simulink model "FullOrderObserver"  (R2024b)
settings: Solver=ode45  StartTime=0.0  StopTime=inf  MaxStep=5e-6  RelTol=1e-3  EnableMultiTasking=on
InitFcn:
  | %电机参数
  | Pe=4000; Ve=380; fe=50;
  | Rs=1.087; Rr=0.788;
  | Ls=0.148; Lr=0.148; Lm=0.140;
  | J=0.0131;FF=0.002985; np=2;
  | %其他参数
  | Ts=5e-6;
  | fs=5000;
  | Udc=540;
  | k=1.5;
undefined symbols (not defined in the file): DiscIntNeverNeededParam, spd
libraries: powerlib_extras x3, spsDCVoltageSourceLib x2, spsAsynchronousMachineSIUnitsLib x1, spsGroundLib x1, simulink x1, spsThreePhaseVIMeasurementLib x1, spsUniversalBridgeLib x1, sps_lib x1
settings Model: Creator=Lenovo  LastModifiedBy=SESA504213
settings SolverCC: AlgebraicLoopSolver=TrustRegion
settings DataIOCC: LimitDataPoints=on  SaveFormat=Array  SignalLoggingSaveFormat=ModelDataLogs  ReturnWorkspaceOutputs=off
settings OptimizationCC: ExpressionDepthLimit=2147483647  LifeSpan=inf
settings DebuggingCC: UnderspecifiedInitializationDetection=Classic  MergeDetectMultiDrivingBlocksExec=none  SolverPrmCheckMsg=warning  FcnCallInpInsideContextMsg=warning  UnconnectedInputMsg=warning  UnconnectedOutputMsg=warning  UnconnectedLineMsg=warning  StateNameClashWarn=warning  SFUnexpectedBacktrackingDiag=warning  SFNoUnconditionalDefaultTransitionDiag=warning  SFExecutionAtInitializationDiag=none  ArithmeticOperatorsInVariantConditions=warning
settings HardwareCC: ProdBitPerPointer=32  ProdBitPerSizeT=32  ProdBitPerPtrDiffT=32  ProdLargestAtomicFloat=None  ProdIntDivRoundTo=Undefined  ProdEndianess=Unspecified  ProdWordSize=32  ProdHWDeviceType=32-bit Generic
settings ModelReferenceCC: EnableRefExpFcnMdlSchedulingChecks=on  PropagateSignalLabelsOutOfModel=off
settings SFSimCC: SimUseLocalCustomCode=off  CustomCodeUndefinedFunction=UseInterfaceOnly
settings RTWCC: RTWUseLocalCustomCode=off  GPUComputeCapability=3.5
settings CodeAppCC: StateflowObjectComments=on
settings GRTTargetCC: TargetLangStandard=C89/C90 (ANSI)  CombineOutputUpdateFcns=off  GRTInterface=on
settings ConfigComp: CovMetricSettings=dw  CovSaveCumulativeToWorkspaceVar=on  CovSaveSingleToWorkspaceVar=on  CovExternalEMLEnable=off

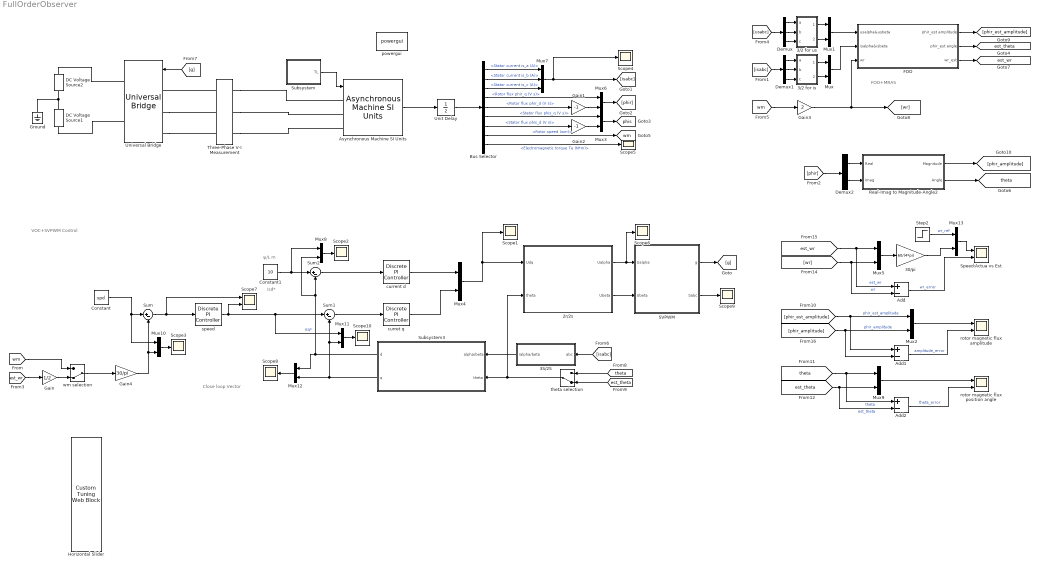
== system FullOrderObserver ==
  note: FOO+MRAS
  note: VOC+SVPWM Control
  note: Close loop Vector
  note: ψ/L m
  note: isd*
  " rotor magnetic flux amplitude" : Scope  NumInputPorts=2
  2r/2s : Subsystem
  3/2 for is : Subsystem
  3/2 for us : Subsystem
  30/pi : Gain  Gain=60/(4*pi)
  3S/2S : Subsystem
  Add : Sum  Inputs=+-
  Add1 : Sum  Inputs=+-
  Add2 : Sum  Inputs=+-
  Asynchronous Machine SI Units : spsAsynchronousMachineSIUnitsLib/Asynchronous Machine SI Units  RotorType=Squirrel-cage  PresetModel=No  MechanicalLoad=Torque Tm  ShowDetailedParameters=on  ReferenceFrame=Stationary  Units=SI  MeasurementBus=off  NominalParameters=[Pe Ve fe]  VoltageRatio=1  Stator=[Rs Ls-Lm]  Rotor=[Rr Lr-Lm]  Cage1=[ 0.022 0.226/377]  Cage2=[ 0.022 0.226/377]  Lm=Lm  Mechanical=[J FF np]  PolePairs=2  InitialConditions=[1 0 0 0 0 0 0 0]  SimulateSaturation=off  Saturation=[14.03593122, 27.81365428, 53.79336849, 72.68890987, 97.98006896, 148.6815601, 215.7428561, 302.9841135, 420.4778367 ; 230, 322, 414, 460, 506, 552, 598, 644, 690]  LoadFlowParameters=1492000  TsPowergui=0  TsBlock=-1  IterativeModel=Forward Euler  IterativeDiscreteModel=Trapezoidal non iterative  Pmec=1.492e+006
      settings: AttributesFormatString=\n
  Bus Selector : BusSelector  OutputSignals=Stator measurements.Stator current is_a (A),Stator measurements.Stator current is_b (A),Stator measurements.Stator current is_c (A),Rotor measurements.Rotor flux phir_q (V s),Rotor measurements.Rotor flux phir_d (V s),Stator measurements.Stator flux phis_q (V s),Stator measurements.Stator flux phis_d (V s),Mechanical.Rotor speed (wm),Mechanical.Electromagnetic torque Te (N*m)
  Constant : Constant  Value=spd
  Constant1 : Constant  Value=10  SampleTime=0
  DC Voltage Source1 : spsDCVoltageSourceLib/DC Voltage Source  Amplitude=Udc/2  Measurements=None
  DC Voltage Source2 : spsDCVoltageSourceLib/DC Voltage Source  Amplitude=Udc/2  Measurements=None
  Demux : Demux  Outputs=3
  Demux1 : Demux  Outputs=3
  Demux2 : Demux  Outputs=2
  FOO : Subsystem
  Gain : Gain  Gain=1/2
  Gain1 : Gain  Gain=-1
  Gain2 : Gain  Gain=-1
  Gain3 : Gain  Gain=2
  Gain4 : Gain  Gain=30/pi
  Ground : spsGroundLib/Ground  LConnTagsString=a
  Horizontal Slider : CustomTuningWebBlock  LabelPosition=Hide  ShowInitialText=on  Configuration="{\"components\":[{\"name\":\"LinearScaleComponent\",\"settings\":{\"bounds\":{\"max\":3000,\"min\":0,\"tickInterval\":\"auto\"},\"internalTickHeightScaleFactor\":0.5,\"labelColor\":[255,255,200],\"labelFont\":{\"font\":\"Arial\",\"fontSize\":12},\"labelOffset\":0.05,\"labelTransparency\":1,\"needleImage\":{\"size\":[596,842],\"src\":\"data:image\\/svg+xml;base64,PD94bWwgdmVyc2lvbj0iMS4wIiBlbmNvZGluZz0idXRmLTgiPz4NCjwhLS0gR2VuZXJhdG9yOiBBZG9iZSBJbGx1c3RyYXRvciAyNS4wLjAsIFNWRyBFeHBvcnQgUGx1Zy1JbiAuIFNWRyBWZXJzaW9uOiA2LjAwIEJ1aWxkIDApICAtLT4NCjxzdmcgdmVyc2lvbj0iMS4xIg0KCSBpZD0ic3ZnOCIgeG1sbnM6Y2M9Imh0dHA6Ly9jcmVhdGl2ZWNvbW1vbnMub3JnL25zIyIgeG1sbnM6ZGM9Imh0dHA6Ly9wdXJsLm9yZy9kYy9lbGVtZW50cy8xLjEvIiB4bWxuczppbmtzY2FwZT0iaHR0cDovL3d3dy5pbmtzY2FwZS5vcmcvbmFtZXNw ...(+2420 chars)\",\"srcOrientation\":\"Right\"},\"needleOffset\":[0.0642123287671233,-0.8044596912521441],\"needleSize\":{\"height\":0.07668067226890757,\"width\":0.4337797619047619},\"position\":[0.03637079831932777,0.2829861111111111,0.6088789682539683,0.9196428571428571],\"referencePoint\":\"auto\",\"scaleColors\":[],\"scaleColorsSize\":0.2,\"scaleDirection\":\"BT\",\"showLabels\":1,\"showMinorTicks\":0,\"showSpanLine\":1,\"showTicks\":1,\"tickColor\":[252,252,197],\"tickTransparency\":1,\"valueBarColor\":[0,114,189],\"valueBarOffset\":-0.27,\"valueBarSize\":0.1,\"valueBarTransparency\":1}},{\"name\":\"BackgroundImageComponent\",\"settings\":{\"image\":{\"size\":[380,101],\"src\":\"data:image\\/svg+xml;base64,PHN2ZyB4bWxucz0iaHR0cDovL3d3dy53My5vcmcvMjAwMC9zdmciIHhtbG5zOnhsaW5rPSJodHRwOi8vd3d3LnczLm9yZy8xOTk5L3hsaW5rIiB2aWV3Qm94PSIwIDAgMzgwIDEwMSI+PGRlZnM+PHN0eWxlPi5jbHMtMXtmaWxsOiMwMDJiNDI7fS5jbHMtMntmaWxsOiM0MjcwODI7fS5jbHMtM3tmaWxsOnVybCgjcmFkaWFsLWdyYWRpZW50KTt9LmNscy00e2ZpbGw6I2M4YzhjODtzdHJva2U6IzAwMDt9PC9zdHlsZT48cmFkaWFsR3JhZGllbnQgaWQ9InJhZGlhbC1ncmFkaWVudCIgY3g9IjE5MCIgY3k9IjUwLjUiIHI9IjI2OS4yMSIgZ3JhZGllbnRVbml0cz0idXNlclNwYWNlT25Vc2UiPjxzdG9wIG9mZnNldD0iMC4wMSIgc3RvcC1jb2xvcj0iIzNlNGY1OCIvPjxzdG9wIG9mZnNldD0iMC4wNiIgc3RvcC1jb2xvcj0iIzQ0NTc2MSIvPjxzdG9wIG9mZnNldD0iMC4xNSIgc3RvcC1jb2xvcj0iIzU1NmE3NiIvPjxzdG9wIG9mZnNldD0iMC4yNSIgc3RvcC1jb2xvcj0iIzZkODg5NSIvPjxzdG9wIG9mZnNldD0iMC4zOCIgc3RvcC1jb2xvcj0iIzhmYjJjMyIvPjxzdG9wIG9mZnNldD0iMC41MiIgc3RvcC1jb2xvcj0iI2I2ZTRmYSIvPjxzdG9wIG9mZnNldD0iMSIgc3RvcC1jb2xvcj0iIzE1NDY1NyIvPjwvcmFkaWFsR3JhZGllbnQ+PC9kZWZzPjxnIGlkPSJmcmFtZSI+PGcgaWQ9IkxheWVyXzIiIGRhdGEtbmFtZT0iTGF5ZXIgMiI+PGcgaWQ9IkxheWVyXzEtMiIgZGF0YS1uYW1lPSJMYXllciAxLTIiPjxyZWN0IGlkPSJyZWN0MTAzNiIgY2xhc3M9ImNscy0xIiB4PSIxMSIgeT0iMTEiIHdpZHRoPSIzNTgiIGhlaWdodD0iNzkiLz48cGF0aCBpZD0icGF0aDEwMzgiIGNsYXNzPSJjbHMtMiIgZD0iTTgsOFY5M0gzNzJWOFpNMzY5LDkwSDExVjExSDM2OVoiLz48cGF0aCBpZD0icGF0aDEwNDAiIGNsYXNzPSJjbHMtMyIgZD0iTTAsMFYxMDFIMzgwVjBaTTM3Miw5M0g4VjhIMzcyWiIvPjwvZz48L2c+PC9nPjxnIGlkPSJ0cmFjayI+PHBhdGggaWQ9InJlY3QxNjExIiBjbGFzcz0iY2xzLTQiIGQ9Ik0zMy4zNywyNi41OUgzNDYuNjNjNCwwLDcuMjUsMi42LDcuMjUsNS44MWgwYzAsMy4yMS0zLjI1LDUuODItNy4yNSw1LjgySDMzLjM3Yy00LDAtNy4yNS0yLjYxLTcuMjUtNS44MmgwQzI2LjEyLDI5LjE5LDI5LjM3LDI2LjU5LDMzLjM3LDI2LjU5WiIvPjwvZz48L3N2Zz4=\",\"srcOrientation\":\"horizontal\"},\"position\":[0,0,1,1],\"scaleMode\":\"0\"}},{\"name\":\"ForegroundImageComponent\",\"settings\":{\"image\":{\"size\":[0,0],\"src\":\"default\",\"srcOrientation\":[]},\"isForeground\":1,\"position\":[0,0,1,1],\"scaleMode\":\"0\"}}],\"settings\":{\"BindingType\":\"param\",\"aspectRatio\":3.7777777777777777,\"backgroundColor\":[0,0,0,\"1\"],\"backgroundOffset\":0,\"backgroundOpacity\":1,\"fixedAspectRatio\":\"on\",\"foregroundColor\":[252,252,196],\"orientation\":\"vertical\",\"showBackgroundColor\":false,\"value\":0,\"version\":\"R2023a\"},\"type\":\"LinearGauge\"}"
  Mux{,1..6,8..13} (13 alike) : Mux  Inputs=2
  Mux7 : Mux  Inputs=3
  Real-Imag to Magnitude-Angle2 : Subsystem
  SVPWM : Subsystem
  Scope{1..6,8..10} (9 alike) : Scope
  Scope7 : Scope  NumInputPorts=2
  Speed:Actua vs Est : Scope  NumInputPorts=2
  Step2 : Step  Before=500  After=1000  SampleTime=0
  Subsystem : Subsystem
  Subsystem3 : Subsystem
  Sum : Sum  Inputs=|+-
  Sum1 : Sum  Inputs=|+-
  Sum2 : Sum  Inputs=|+-
  Three-Phase V-I Measurement : spsThreePhaseVIMeasurementLib/Three-Phase V-I Measurement  VoltageMeasurement=phase-to-ground  SetLabelV=on  LabelV=usabc  Vpu=off  VpuLL=off  CurrentMeasurement=no  SetLabelI=off  LabelI=Iabc  Ipu=off  Pbase=100e6  Vbase=500e3  OutputType=Complex  PhasorSimulation=off  PSBequivalent=0
  Unit Delay : UnitDelay  SampleTime=-1
  Universal Bridge : spsUniversalBridgeLib/Universal Bridge  Arms=3  SnubberResistance=1e5  SnubberCapacitance=inf  Device=IGBT / Diodes  Ron=1e-3  Lon=0  ForwardVoltages="[  0  0  ]"  ForwardVoltage=0  GTOparameters=[ 10e-6 , 20e-6 ]  IGBTparameters=[ 1e-6 , 2e-6]  Measurements=Device voltages  Measurements_2=None  converterType=Rectifier
  current d : powerlib_extras/Discrete  Control Blocks/Discrete PI Controller  Kp=15*15  Ki=600*2  Par_Limits=[310*1.5 -310*1.5]  Init=0  Ts=-1
  curret q : powerlib_extras/Discrete  Control Blocks/Discrete PI Controller  Kp=15*15  Ki=600*2  Par_Limits=[310*1.5 -310*1.5]  Init=0  Ts=-1
  powergui : sps_lib/powergui  Priority=1  SimulationMode=Discrete  SampleTime=5e-6  frequency=60  Iterations=50  frequencyindice=50  Pbase=100e6  ErrMax=1e-4  UnitsV=kV  UnitsW=MW  buscounter=0  FunctionMessages=off  echomessages=off  EnableUseOfTLC=off  CurrentSourceSwitches=off  DisableSnubberDevices=off  DisableRonSwitches=off  DisableVfSwitches=off  DisplayEquations=off  AutomaticDiscreteSolvers=off  SolverType=Tustin/Backward Euler (TBE)  Interpol=off  ExternalGateDelay=off  methode=off  Ts=0  x0status=blocks  SPID=off  SwTol=0  HookPort=off  NonlinearTolerance=1e-4  nMaxIteration=100  ContinueOnMaxIteration=off  RestoreLinks=warning  ResistiveCurrentMeasurement=off  Frange=[0:2:500]  Ylog=off  Xlog=on  ShowGrid=off  save=off  variable=ZData  structure=0  ZoomFFT=off  StartTime=0.0  cycles=1  DisplayStyle=1  fundamental=60  FreqAxis=off  MaxFrequency=1000  frequencyindicesteady=1  RmsSteady=1  display=off
  "rotor magnetic flux position angle " : Scope  NumInputPorts=2
  speed : powerlib_extras/Discrete  Control Blocks/Discrete PI Controller  Kp=0.4  Ki=15  Par_Limits=[30 -30]  Init=0  Ts=-1
  theta selection : ManualSwitch  CurrentSetting=0
  wm selection : ManualSwitch  CurrentSetting=0
  tag scope: est_theta=global, est_wr=global, phis=global, theta=global, wm=global
  wires:
  Bus Selector/1 -> Mux7/1  "<Stator current is_a (A)>"
  Bus Selector/2 -> Mux7/2  "<Stator current is_b (A)>"
  Bus Selector/3 -> Mux7/3  "<Stator current is_c (A)>"
  Gain2/1 -> Mux3/2
  Mux2/1 -> " rotor magnetic flux amplitude"/1
  Mux5/1 -> 30/pi/1
  Demux2/1 -> Real-Imag to Magnitude-Angle2/1(Real)
  Demux2/2 -> Real-Imag to Magnitude-Angle2/2(Imag)
  Bus Selector/7 -> Gain2/1  "<Stator flux phis_d (V s)>"
  Bus Selector/6 -> Mux3/1  "<Stator flux phis_q (V s)>"
  [isabc] -> Demux1/1
  Demux1/1 -> 3/2 for is/1(a)
  Demux1/2 -> 3/2 for is/2(b)
  Demux1/3 -> 3/2 for is/3(c)
  3/2 for is/1(alpha) -> Mux/1
  3/2 for is/2(beta) -> Mux/2
  Gain1/1 -> Mux6/2
  Bus Selector/5 -> Gain1/1  "<Rotor flux phir_d (V s)>"
  Bus Selector/4 -> Mux6/1  "<Rotor flux phir_q (V s)>"
  Mux6/1 -> [phir]
  Mux3/1 -> [phis]
  [usabc] -> Demux/1
  Demux/1 -> 3/2 for us/1(a)
  Demux/2 -> 3/2 for us/2(b)
  Demux/3 -> 3/2 for us/3(c)
  3/2 for us/1(alpha) -> Mux1/1
  3/2 for us/2(beta) -> Mux1/2
  Mux1/1 -> FOO/1(usalpha&usbeta)
  Mux/1 -> FOO/2(isalpha&isbeta)
  Bus Selector/8 -> [wm]  "<Rotor speed (wm)>"
  [wm] -> Gain3/1
  Mux9/1 -> "rotor magnetic flux position angle "/1
  [phir] -> Demux2/1
  FOO/2(phir_est angle) -> [est_theta]
  Gain3/1 -> [wr], FOO/3("wr ")
  Bus Selector/9 -> Scope5/1  "<Electromagnetic torque Te (N*m)>"
  FOO/3(wr_est) -> [est_wr]
  30/pi/1 -> Mux13/2
  Real-Imag to Magnitude-Angle2/2(Angle) -> [theta]
  Mux7/1 -> [isabc], Scope4/1
  SVPWM/1(g) -> [g]
  [g] -> Universal Bridge/1
  [wm] -> wm selection/1
  [theta] -> theta selection/1
  [est_theta] -> theta selection/2
  Asynchronous Machine SI Units/1 -> Unit Delay/1
  Unit Delay/1 -> Bus Selector/1
  Gain/1 -> wm selection/2
  [est_wr] -> Gain/1
  wm selection/1 -> Gain4/1
  theta selection/1 -> Subsystem3/2(theta), 2r/2s/2(theta)
  SVPWM/2(Sabc) -> Scope9/1
  speed/1 -> Sum1/1, Mux11/1, Scope7/2  "isq*"
  Constant/1 -> Mux10/1, Sum/1
  Sum/1 -> Scope7/1, speed/1
  Sum2/1 -> current d/1
  curret q/1 -> Mux4/2
  current d/1 -> Mux4/1
  Mux11/1 -> Scope10/1
  Mux10/1 -> Scope3/1
  Mux12/1 -> Scope8/1
  Mux8/1 -> Scope2/1
  Gain4/1 -> Mux10/2, Sum/2
  Sum1/1 -> curret q/1
  Mux4/1 -> Scope1/1, 2r/2s/1(Udq)
  2r/2s/2(Ubeta) -> SVPWM/2(Ubeta)
  2r/2s/1(Ualpha) -> Scope6/1, SVPWM/1(Ualpha)
  Subsystem3/2(q) -> Sum1/2, Mux11/2, Mux12/2
  Subsystem3/1(d) -> Mux12/1, Sum2/2, Mux8/2
  3S/2S/1(ialpha/beta) -> Subsystem3/1(alpha/beta)
  [isabc] -> 3S/2S/1(abc)
  Constant1/1 -> Mux8/1, Sum2/1
  Add/1 -> Speed:Actua vs Est/2  "wr_error"
  [est_wr] -> Mux5/1, Add/1  "est_wr"
  [theta] -> Mux9/1, Add2/1  "theta"
  [est_theta] -> Mux9/2, Add2/2  "est_theta"
  [wr] -> Mux5/2, Add/2  "wr"
  FOO/1(phir_est amplitude) -> [phir_est_amplitude]
  Real-Imag to Magnitude-Angle2/1(Magnitude) -> [phir_amplitude]
  [phir_amplitude] -> Mux2/2, Add1/2  "phir_amplitude"
  Add1/1 -> " rotor magnetic flux amplitude"/2  "amplitude_error"
  Add2/1 -> "rotor magnetic flux position angle "/2  "theta_error"
  Step2/1 -> Mux13/1  "wr_ref"
  Mux13/1 -> Speed:Actua vs Est/1
  [phir_est_amplitude] -> Add1/1, Mux2/1  "phir_est_amplitude"
  Subsystem/1(TL) -> Asynchronous Machine SI Units/1
  connections:
  DC Voltage Source1/RConn1 -- Ground/LConn1 -- DC Voltage Source2/LConn1
  DC Voltage Source1/LConn1 -- Universal Bridge/RConn2
  Three-Phase V-I Measurement/RConn2 -- Asynchronous Machine SI Units/LConn2
  Three-Phase V-I Measurement/RConn1 -- Asynchronous Machine SI Units/LConn1
  Three-Phase V-I Measurement/LConn1 -- Universal Bridge/LConn1
  Universal Bridge/LConn2 -- Three-Phase V-I Measurement/LConn2
  Universal Bridge/LConn3 -- Three-Phase V-I Measurement/LConn3
  Three-Phase V-I Measurement/RConn3 -- Asynchronous Machine SI Units/LConn3
  DC Voltage Source2/RConn1 -- Universal Bridge/RConn1

== system FullOrderObserver/2r//2s ==
  Udq : Inport
  theta : Inport  Port=2
  Demux : Demux  Outputs=2
  Mux1 : Mux  Inputs=2
  Product{,1..3} (4 alike) : Product  RndMeth=Zero
  Scope1 : Scope
  Sum : Sum  Inputs=|+-
  Sum1 : Sum  Inputs=|++
  Trigonometric Function : Trigonometry
  Trigonometric Function1 : Trigonometry  Operator=cos
  Ualpha : Outport
  Ubeta : Outport  Port=2
  wires:
  Udq/1 -> Demux/1
  Product/1 -> Sum/1
  Product1/1 -> Sum/2
  Product2/1 -> Sum1/1
  Product3/1 -> Sum1/2
  Sum/1 -> Ualpha/1, Mux1/1
  Sum1/1 -> Ubeta/1, Mux1/2
  Demux/1 -> Product/1, Product2/1
  Trigonometric Function1/1 -> Product/2, Product3/2
  Demux/2 -> Product1/1, Product3/1
  Trigonometric Function/1 -> Product1/2, Product2/2
  theta/1 -> Trigonometric Function/1, Trigonometric Function1/1
  Mux1/1 -> Scope1/1

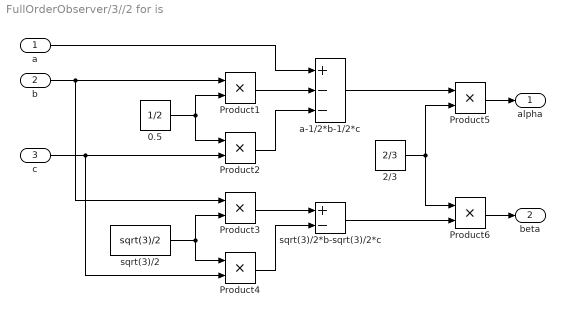
== system FullOrderObserver/3//2 for is ==
  a : Inport
  b : Inport  Port=2
  c : Inport  Port=3
  0.5 : Constant  Value=1/2
  2/3 : Constant  Value=2/3
  Product{1..6} (6 alike) : Product  RndMeth=Zero
  a-1/2*b-1/2*c : Sum  Inputs=+--
  sqrt(3)/2 : Constant  Value=sqrt(3)/2
  sqrt(3)/2*b-sqrt(3)/2*c : Sum  Inputs=+-
  alpha : Outport
  beta : Outport  Port=2
  wires:
  0.5/1 -> Product1/2, Product2/1
  sqrt(3)/2/1 -> Product3/2, Product4/1
  b/1 -> Product1/1, Product3/1
  c/1 -> Product2/2, Product4/2
  Product1/1 -> a-1/2*b-1/2*c/2
  Product2/1 -> a-1/2*b-1/2*c/3
  a/1 -> a-1/2*b-1/2*c/1
  Product3/1 -> sqrt(3)/2*b-sqrt(3)/2*c/1
  Product4/1 -> sqrt(3)/2*b-sqrt(3)/2*c/2
  a-1/2*b-1/2*c/1 -> Product5/1
  2/3/1 -> Product5/2, Product6/1
  sqrt(3)/2*b-sqrt(3)/2*c/1 -> Product6/2
  Product5/1 -> alpha/1
  Product6/1 -> beta/1

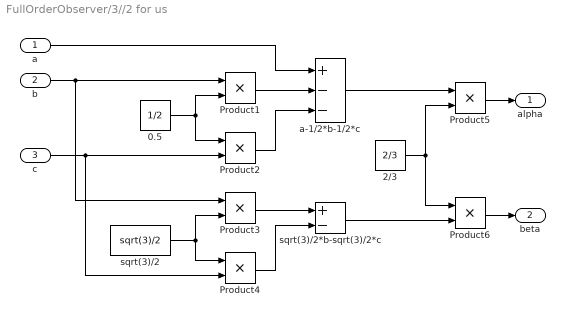
== system FullOrderObserver/3//2 for us ==
  a : Inport
  b : Inport  Port=2
  c : Inport  Port=3
  0.5 : Constant  Value=1/2
  2/3 : Constant  Value=2/3
  Product{1..6} (6 alike) : Product  RndMeth=Zero
  a-1/2*b-1/2*c : Sum  Inputs=+--
  sqrt(3)/2 : Constant  Value=sqrt(3)/2
  sqrt(3)/2*b-sqrt(3)/2*c : Sum  Inputs=+-
  alpha : Outport
  beta : Outport  Port=2
  wires:
  Product6/1 -> beta/1
  Product5/1 -> alpha/1
  sqrt(3)/2*b-sqrt(3)/2*c/1 -> Product6/2
  2/3/1 -> Product6/1, Product5/2
  a-1/2*b-1/2*c/1 -> Product5/1
  Product4/1 -> sqrt(3)/2*b-sqrt(3)/2*c/2
  Product3/1 -> sqrt(3)/2*b-sqrt(3)/2*c/1
  a/1 -> a-1/2*b-1/2*c/1
  Product2/1 -> a-1/2*b-1/2*c/3
  Product1/1 -> a-1/2*b-1/2*c/2
  c/1 -> Product4/2, Product2/2
  b/1 -> Product3/1, Product1/1
  sqrt(3)/2/1 -> Product4/1, Product3/2
  0.5/1 -> Product2/1, Product1/2

== system FullOrderObserver/3S//2S ==
  abc : Inport
  Demux : Demux  Outputs=3
  Gai2 : Gain  Gain=-1/2
  Gain1 : Gain  Gain=-1/2
  Gain3 : Gain  Gain=(sqrt(3))/2
  Gain4 : Gain  Gain=(sqrt(3))/2
  Gain5 : Gain  Gain=2/3
  Gain6 : Gain  Gain=2/3
  Mux3 : Mux  Inputs=2
  Sum : Sum  Inputs=|++
  Sum1 : Sum  Inputs=|++
  Sum2 : Sum  Inputs=|-+
  ialpha/beta : Outport
  wires:
  Mux3/1 -> ialpha/beta/1
  Gain5/1 -> Mux3/1
  Gain6/1 -> Mux3/2
  Demux/3 -> Gain4/1, Gai2/1
  Demux/2 -> Gain3/1, Gain1/1
  Demux/1 -> Sum/1
  Sum2/1 -> Gain6/1
  Sum1/1 -> Gain5/1
  Gain3/1 -> Sum2/2
  Gain4/1 -> Sum2/1
  Sum/1 -> Sum1/1
  Gai2/1 -> Sum1/2
  Gain1/1 -> Sum/2
  abc/1 -> Demux/1

== system FullOrderObserver/FOO ==
  usalpha&usbeta : Inport
  isalpha&isbeta : Inport  Port=2
  "wr " : Inport  Port=3
  " Speed-Adaptation" : Subsystem  mask{Kp=15, Ki=5000}
      mask prompts: Kp "Kp="; Ki "Ki="
  Demux : Demux  Outputs=2
  Demux1 : Demux  Outputs=2
  Real-Imag to Magnitude-Angle : Subsystem
  full order flux observer : Subsystem
  wr selection : ManualSwitch  CurrentSetting=0
  phir_est amplitude : Outport
  phir_est angle : Outport  Port=2
  wr_est : Outport  Port=3
  wires:
  " Speed-Adaptation"/1(wr_est) -> wr_est/1, wr selection/2
  full order flux observer/3(phiralpha_est2) -> " Speed-Adaptation"/5(phiralpha_est), full order flux observer/3(phiralpha_est), Real-Imag to Magnitude-Angle/1(Real)
  wr selection/1 -> full order flux observer/9(wr)
  full order flux observer/2(phisbeta_est2) -> full order flux observer/2(phisbeta_est)
  full order flux observer/6(isbeta_est) -> " Speed-Adaptation"/4(isbeta_est)
  full order flux observer/1(phisalpha_est2) -> full order flux observer/1(phisalpha_est)
  full order flux observer/4(phirbeta_est2) -> " Speed-Adaptation"/6(phirbeta_est), full order flux observer/4(phirbeta_est), Real-Imag to Magnitude-Angle/2(Imag)
  full order flux observer/5(isalpha_est) -> " Speed-Adaptation"/3(isalpha_est)
  "wr "/1 -> wr selection/1
  Demux1/2 -> " Speed-Adaptation"/2(isbeta), full order flux observer/8(isbeta)
  Demux/2 -> full order flux observer/6(usbeta)
  Real-Imag to Magnitude-Angle/2(Angle) -> phir_est angle/1
  Real-Imag to Magnitude-Angle/1(Magnitude) -> phir_est amplitude/1
  Demux/1 -> full order flux observer/5(usalpha)
  usalpha&usbeta/1 -> Demux/1
  Demux1/1 -> " Speed-Adaptation"/1(isalpha), full order flux observer/7(isalpha)
  isalpha&isbeta/1 -> Demux1/1

== system FullOrderObserver/Real-Imag to Magnitude-Angle2 ==
  Real : Inport
  Imag : Inport  Port=2
  2*pi : Constant  Value=2*pi  VectorParams1D=off
  Add : Sum
  Complex to Magnitude-Angle : ComplexToMagnitudeAngle
  Real-Imag to Complex : RealImagToComplex
  Switch : Switch  Criteria=u2 > Threshold  SaturateOnIntegerOverflow=off  InputSameDT=off
  Magnitude : Outport
  Angle : Outport  Port=2
  wires:
  Complex to Magnitude-Angle/2 -> Switch/1, Add/1, Switch/2
  Real-Imag to Complex/1 -> Complex to Magnitude-Angle/1
  Imag/1 -> Real-Imag to Complex/2
  2*pi/1 -> Add/2
  Add/1 -> Switch/3
  Real/1 -> Real-Imag to Complex/1
  Switch/1 -> Angle/1
  Complex to Magnitude-Angle/1 -> Magnitude/1

== system FullOrderObserver/SVPWM ==
  Ualpha : Inport
  Ubeta : Inport  Port=2
  Gain1 : Gain  Gain=2500
  Pulse : Subsystem
  SVPWM : Subsystem
  Scope4 : Scope
  Ts : Constant  Value=1/fs
  Udc : Constant  Value=Udc
  g : Outport
  Sabc : Outport  Port=2
  tag scope: N=global
  wires:
  SVPWM/4(N4) -> [N]
  Pulse/2(Sabc) -> Sabc/1
  Udc/1 -> SVPWM/3(Udc)
  Pulse/1(Pulses) -> g/1
  Ubeta/1 -> SVPWM/2(Ubeta)
  Ualpha/1 -> SVPWM/1(Ualfa)
  Ts/1 -> SVPWM/4(Ts)
  Gain1/1 -> Scope4/1
  SVPWM/1(Tcm1) -> Pulse/1(tcm1), Gain1/1
  SVPWM/2(Tcm2) -> Pulse/2(tcm2)
  SVPWM/3(Tcm3) -> Pulse/3(tcm3)

== system FullOrderObserver/Subsystem ==
  Constant : Constant  Value=0
  Manual Switch : ManualSwitch
  Step : Step  Time=0.5  After=2  SampleTime=0
  TL : Outport  VectorParamsAs1DForOutWhenUnconnected=off
  wires:
  Step/1 -> Manual Switch/2
  Constant/1 -> Manual Switch/1
  Manual Switch/1 -> TL/1

== system FullOrderObserver/Subsystem3 ==
  alpha/beta : Inport
  theta : Inport  Port=2
  Demux1 : Demux  Outputs=2
  Product{,1..3} (4 alike) : Product  RndMeth=Zero
  Sum : Sum  Inputs=|++
  Sum1 : Sum  Inputs=|-+
  Trigonometric Function : Trigonometry
  Trigonometric Function1 : Trigonometry  Operator=cos
  d : Outport
  q : Outport  Port=2
  wires:
  alpha/beta/1 -> Demux1/1
  Demux1/1 -> Product2/1, Product/1
  Demux1/2 -> Product3/1, Product1/1
  Sum1/1 -> q/1
  Sum/1 -> d/1
  Product3/1 -> Sum1/2
  Product2/1 -> Sum1/1
  Product1/1 -> Sum/2
  Product/1 -> Sum/1
  Trigonometric Function/1 -> Product2/2, Product1/2
  Trigonometric Function1/1 -> Product3/2, Product/2
  theta/1 -> Trigonometric Function1/1, Trigonometric Function/1

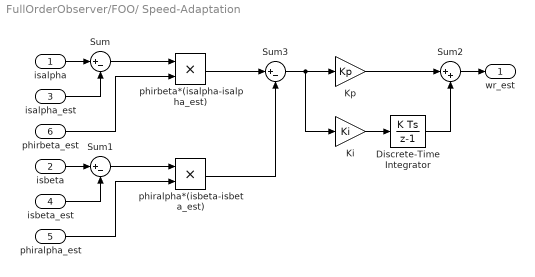
== system FullOrderObserver/FOO/ Speed-Adaptation ==
  isalpha : Inport
  isbeta : Inport  Port=2
  isalpha_est : Inport  Port=3
  isbeta_est : Inport  Port=4
  phiralpha_est : Inport  Port=5
  phirbeta_est : Inport  Port=6
  Discrete-Time Integrator : DiscreteIntegrator  SampleTime=Ts  ICPrevOutput=DiscIntNeverNeededParam  ICPrevScaledInput=DiscIntNeverNeededParam
  Ki : Gain  Gain=Ki
  Kp : Gain  Gain=Kp
  Sum : Sum  Inputs=|+-
  Sum1 : Sum  Inputs=|+-
  Sum2 : Sum  Inputs=|++
  Sum3 : Sum  Inputs=|+-
  phiralpha*(isbeta-isbeta_est) : Product
  phirbeta*(isalpha-isalpha_est) : Product
  wr_est : Outport
  wires:
  Discrete-Time Integrator/1 -> Sum2/2
  Sum/1 -> phirbeta*(isalpha-isalpha_est)/1
  Sum3/1 -> Ki/1, Kp/1
  phiralpha_est/1 -> phiralpha*(isbeta-isbeta_est)/2
  isalpha/1 -> Sum/1
  Sum2/1 -> wr_est/1
  isbeta/1 -> Sum1/1
  phirbeta_est/1 -> phirbeta*(isalpha-isalpha_est)/2
  Sum1/1 -> phiralpha*(isbeta-isbeta_est)/1
  Kp/1 -> Sum2/1
  isalpha_est/1 -> Sum/2
  isbeta_est/1 -> Sum1/2
  phirbeta*(isalpha-isalpha_est)/1 -> Sum3/1
  phiralpha*(isbeta-isbeta_est)/1 -> Sum3/2
  Ki/1 -> Discrete-Time Integrator/1

== system FullOrderObserver/FOO/Real-Imag to Magnitude-Angle ==
  Real : Inport
  Imag : Inport  Port=2
  2*pi : Constant  Value=2*pi  VectorParams1D=off
  Add : Sum
  Complex to Magnitude-Angle : ComplexToMagnitudeAngle
  Real-Imag to Complex : RealImagToComplex
  Switch : Switch  Criteria=u2 > Threshold  SaturateOnIntegerOverflow=off  InputSameDT=off
  Magnitude : Outport
  Angle : Outport  Port=2
  wires:
  Complex to Magnitude-Angle/2 -> Switch/1, Add/1, Switch/2
  Real-Imag to Complex/1 -> Complex to Magnitude-Angle/1
  Imag/1 -> Real-Imag to Complex/2
  2*pi/1 -> Add/2
  Add/1 -> Switch/3
  Real/1 -> Real-Imag to Complex/1
  Switch/1 -> Angle/1
  Complex to Magnitude-Angle/1 -> Magnitude/1

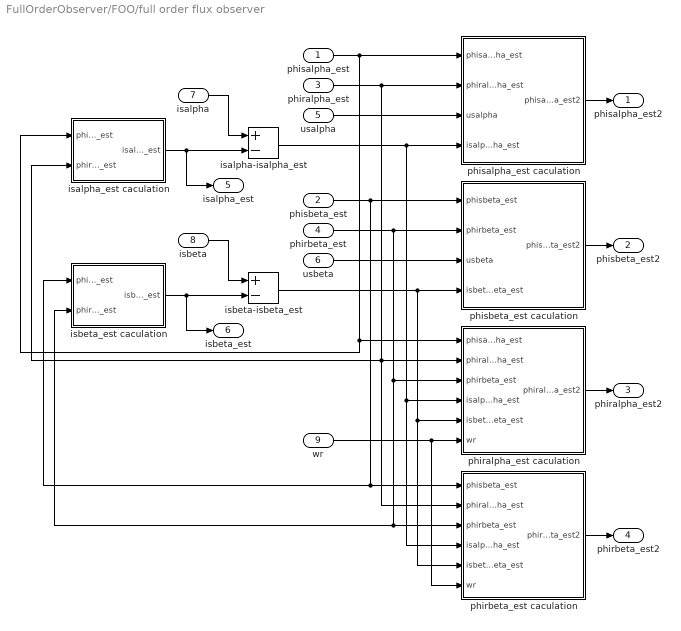
== system FullOrderObserver/FOO/full order flux observer ==
  phisalpha_est : Inport
  phisbeta_est : Inport  Port=2
  phiralpha_est : Inport  Port=3
  phirbeta_est : Inport  Port=4
  usalpha : Inport  Port=5
  usbeta : Inport  Port=6
  isalpha : Inport  Port=7
  isbeta : Inport  Port=8
  wr : Inport  Port=9
  isalpha-isalpha_est : Sum  Inputs=+-
  isalpha_est caculation : Subsystem
  isbeta-isbeta_est : Sum  Inputs=+-
  isbeta_est caculation : Subsystem
  phiralpha_est caculation : Subsystem
  phirbeta_est caculation : Subsystem
  phisalpha_est caculation : Subsystem
  phisbeta_est caculation : Subsystem
  phisalpha_est2 : Outport
  phisbeta_est2 : Outport  Port=2
  phiralpha_est2 : Outport  Port=3
  phirbeta_est2 : Outport  Port=4
  isalpha_est : Outport  Port=5
  isbeta_est : Outport  Port=6
  wires:
  isalpha_est caculation/1(isalpha_est) -> isalpha_est/1, isalpha-isalpha_est/2
  phisalpha_est/1 -> phisalpha_est caculation/1(phisalpha_est), isalpha_est caculation/1(phisalpha_est), phiralpha_est caculation/1(phisalpha_est)
  phirbeta_est/1 -> phisbeta_est caculation/2(phirbeta_est), phiralpha_est caculation/3(phirbeta_est), phirbeta_est caculation/3(phirbeta_est), isbeta_est caculation/2(phirbeta_est)
  usbeta/1 -> phisbeta_est caculation/3(usbeta)
  usalpha/1 -> phisalpha_est caculation/3(usalpha)
  phisbeta_est/1 -> phisbeta_est caculation/1(phisbeta_est), phirbeta_est caculation/1(phisbeta_est), isbeta_est caculation/1(phisbeta_est)
  phirbeta_est caculation/1(phirbeta_est2) -> phirbeta_est2/1
  phisbeta_est caculation/1(phisbeta_est2) -> phisbeta_est2/1
  phiralpha_est/1 -> phisalpha_est caculation/2(phiralpha_est), isalpha_est caculation/2(phiralpha_est), phiralpha_est caculation/2(phiralpha_est), phirbeta_est caculation/2(phiralpha_est)
  isalpha/1 -> isalpha-isalpha_est/1
  phiralpha_est caculation/1(phiralpha_est2) -> phiralpha_est2/1
  wr/1 -> phirbeta_est caculation/6(wr), phiralpha_est caculation/6(wr)
  isbeta/1 -> isbeta-isbeta_est/1
  phisalpha_est caculation/1(phisalpha_est2) -> phisalpha_est2/1
  isbeta_est caculation/1(isbeta_est) -> isbeta_est/1, isbeta-isbeta_est/2
  isalpha-isalpha_est/1 -> phisalpha_est caculation/4(isalpha-isalpha_est), phirbeta_est caculation/4(isalpha-isalpha_est), phiralpha_est caculation/4(isalpha-isalpha_est)
  isbeta-isbeta_est/1 -> phirbeta_est caculation/5(isbeta-isbeta_est), phiralpha_est caculation/5(isbeta-isbeta_est), phisbeta_est caculation/4(isbeta-isbeta_est)

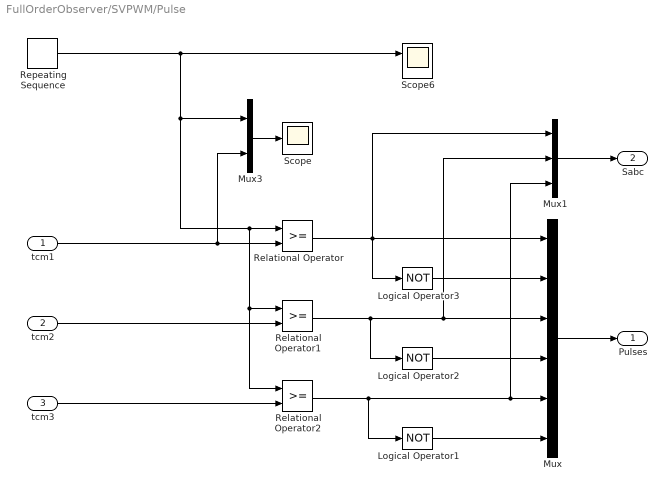
== system FullOrderObserver/SVPWM/Pulse ==
  tcm1 : Inport
  tcm2 : Inport  Port=2
  tcm3 : Inport  Port=3
  Logical Operator1 : Logic  Operator=NOT  AllPortsSameDT=off  OutDataTypeStr=boolean
  Logical Operator2 : Logic  Operator=NOT  AllPortsSameDT=off  OutDataTypeStr=boolean
  Logical Operator3 : Logic  Operator=NOT  AllPortsSameDT=off  OutDataTypeStr=boolean
  Mux : Mux  Inputs=6
  Mux1 : Mux  Inputs=3
  Mux3 : Mux  Inputs=2
  Relational Operator : RelationalOperator  OutDataTypeStr=boolean  InputSameDT=off
  Relational Operator1 : RelationalOperator  OutDataTypeStr=boolean  InputSameDT=off
  Relational Operator2 : RelationalOperator  OutDataTypeStr=boolean  InputSameDT=off
  Repeating Sequence : simulink/Sources/Repeating Sequence  rep_seq_t=[0 0.5 1 ]/fs  rep_seq_y=[0 0.5 0]/fs
  Scope : Scope
  Scope6 : Scope  NumInputPorts=2
  Pulses : Outport
  Sabc : Outport  Port=2
  wires:
  Mux/1 -> Pulses/1
  Relational Operator/1 -> Mux1/1, Mux/1, Logical Operator3/1
  Logical Operator3/1 -> Mux/2
  Relational Operator1/1 -> Mux1/2, Mux/3, Logical Operator2/1
  Logical Operator2/1 -> Mux/4
  Relational Operator2/1 -> Mux1/3, Mux/5, Logical Operator1/1
  Logical Operator1/1 -> Mux/6
  Mux3/1 -> Scope/1
  Mux1/1 -> Sabc/1
  Repeating Sequence/1 -> Mux3/1, Relational Operator1/1, Relational Operator2/1, Relational Operator/1, Scope6/1
  tcm1/1 -> Relational Operator/2, Mux3/2
  tcm2/1 -> Relational Operator1/2
  tcm3/1 -> Relational Operator2/2

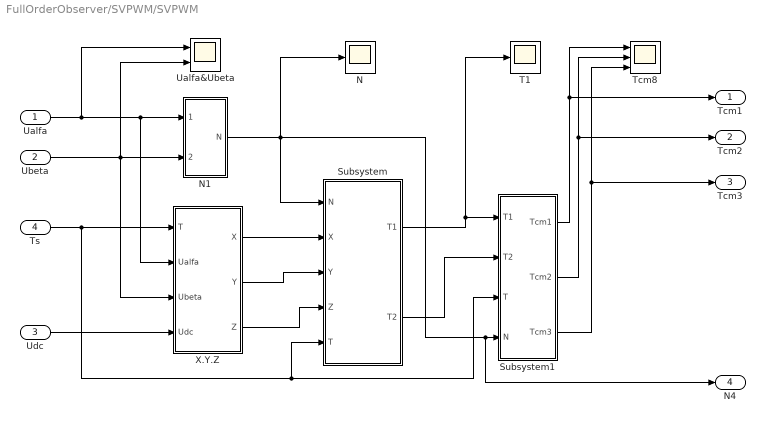
== system FullOrderObserver/SVPWM/SVPWM ==
  Ualfa : Inport
  Ubeta : Inport  Port=2
  Udc : Inport  Port=3
  Ts : Inport  Port=4
  N : Scope
  N1 : Subsystem
  Subsystem : Subsystem
  Subsystem1 : Subsystem
  T1 : Scope
  Tcm8 : Scope  NumInputPorts=3
  Ualfa&Ubeta : Scope  NumInputPorts=2
  X.Y.Z : Subsystem
  Tcm1 : Outport
  Tcm2 : Outport  Port=2
  Tcm3 : Outport  Port=3
  N4 : Outport  Port=4
  wires:
  N1/1(N) -> Subsystem/1(N), N4/1, Subsystem1/4(N), N/1
  X.Y.Z/1(X) -> Subsystem/2(X)
  X.Y.Z/2(Y) -> Subsystem/3(Y)
  X.Y.Z/3(Z) -> Subsystem/4(Z)
  Subsystem1/1(Tcm1) -> Tcm1/1, Tcm8/1
  Subsystem1/2(Tcm2) -> Tcm2/1, Tcm8/2
  Subsystem1/3(Tcm3) -> Tcm3/1, Tcm8/3
  Ualfa/1 -> X.Y.Z/2(Ualfa), N1/1(Ualfa), Ualfa&Ubeta/1
  Subsystem/1(T1) -> Subsystem1/1(T1), T1/1
  Subsystem/2(T2) -> Subsystem1/2(T2)
  Ubeta/1 -> Ualfa&Ubeta/2, X.Y.Z/3(Ubeta), N1/2(Ubeta)
  Udc/1 -> X.Y.Z/4(Udc)
  Ts/1 -> Subsystem1/3(T), Subsystem/5(T), X.Y.Z/1(T)

== system FullOrderObserver/FOO/full order flux observer/isalpha_est caculation ==
  phisalpha_est : Inport
  phiralpha_est : Inport  Port=2
  add : Sum
  c11 : Constant  Value=Lr/(Ls*Lr-Lm*Lm)
  c11*phisalpha_est : Product
  c13 : Constant  Value=-Lm/(Ls*Lr-Lm*Lm)
  c13*phiralpha_est : Product
  isalpha_est : Outport
  wires:
  phiralpha_est/1 -> c13*phiralpha_est/2
  add/1 -> isalpha_est/1
  c11*phisalpha_est/1 -> add/1
  c13*phiralpha_est/1 -> add/2
  phisalpha_est/1 -> c11*phisalpha_est/2
  c11/1 -> c11*phisalpha_est/1
  c13/1 -> c13*phiralpha_est/1

== system FullOrderObserver/FOO/full order flux observer/isbeta_est caculation ==
  phisbeta_est : Inport
  phirbeta_est : Inport  Port=2
  add : Sum
  c11 : Constant  Value=Lr/(Ls*Lr-Lm*Lm)
  c11*phisbeta_est : Product
  c13 : Constant  Value=-Lm/(Ls*Lr-Lm*Lm)
  c13*phirbeta_est : Product
  isbeta_est : Outport
  wires:
  c13/1 -> c13*phirbeta_est/1
  c11/1 -> c11*phisbeta_est/1
  phisbeta_est/1 -> c11*phisbeta_est/2
  c13*phirbeta_est/1 -> add/2
  c11*phisbeta_est/1 -> add/1
  add/1 -> isbeta_est/1
  phirbeta_est/1 -> c13*phirbeta_est/2

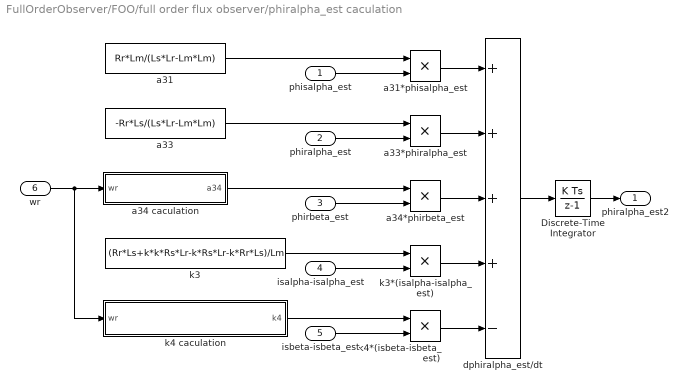
== system FullOrderObserver/FOO/full order flux observer/phiralpha_est caculation ==
  phisalpha_est : Inport
  phiralpha_est : Inport  Port=2
  phirbeta_est : Inport  Port=3
  isalpha-isalpha_est : Inport  Port=4
  isbeta-isbeta_est : Inport  Port=5
  wr : Inport  Port=6
  Discrete-Time Integrator : DiscreteIntegrator  SampleTime=Ts  ICPrevOutput=DiscIntNeverNeededParam  ICPrevScaledInput=DiscIntNeverNeededParam
  a31 : Constant  Value=Rr*Lm/(Ls*Lr-Lm*Lm)
  a31*phisalpha_est : Product
  a33 : Constant  Value=-Rr*Ls/(Ls*Lr-Lm*Lm)
  a33*phiralpha_est : Product
  a34 caculation : Subsystem
  a34*phirbeta_est : Product
  dphiralpha_est/dt : Sum  Inputs=++++-
  k3 : Constant  Value=(Rr*Ls+k*k*Rs*Lr-k*Rs*Lr-k*Rr*Ls)/Lm
  k3*(isalpha-isalpha_est) : Product
  k4 caculation : Subsystem
  k4*(isbeta-isbeta_est) : Product
  phiralpha_est2 : Outport
  wires:
  k3/1 -> k3*(isalpha-isalpha_est)/1
  phisalpha_est/1 -> a31*phisalpha_est/2
  isalpha-isalpha_est/1 -> k3*(isalpha-isalpha_est)/2
  phiralpha_est/1 -> a33*phiralpha_est/2
  Discrete-Time Integrator/1 -> phiralpha_est2/1
  a33*phiralpha_est/1 -> dphiralpha_est/dt/2
  k3*(isalpha-isalpha_est)/1 -> dphiralpha_est/dt/4
  a33/1 -> a33*phiralpha_est/1
  a31*phisalpha_est/1 -> dphiralpha_est/dt/1
  a31/1 -> a31*phisalpha_est/1
  k4 caculation/1(k4) -> k4*(isbeta-isbeta_est)/1
  isbeta-isbeta_est/1 -> k4*(isbeta-isbeta_est)/2
  k4*(isbeta-isbeta_est)/1 -> dphiralpha_est/dt/5
  dphiralpha_est/dt/1 -> Discrete-Time Integrator/1
  wr/1 -> k4 caculation/1(wr), a34 caculation/1(wr)
  a34*phirbeta_est/1 -> dphiralpha_est/dt/3
  a34 caculation/1(a34) -> a34*phirbeta_est/1
  phirbeta_est/1 -> a34*phirbeta_est/2

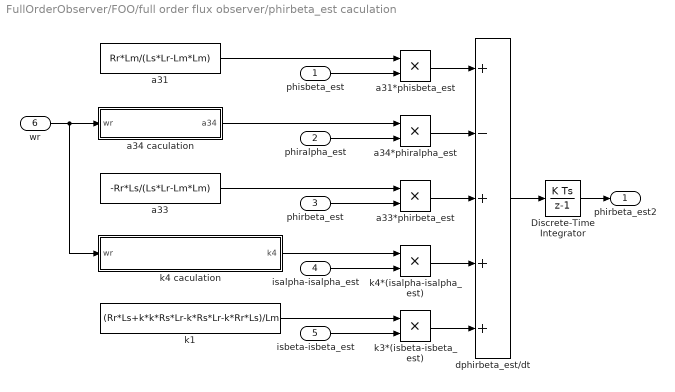
== system FullOrderObserver/FOO/full order flux observer/phirbeta_est caculation ==
  phisbeta_est : Inport
  phiralpha_est : Inport  Port=2
  phirbeta_est : Inport  Port=3
  isalpha-isalpha_est : Inport  Port=4
  isbeta-isbeta_est : Inport  Port=5
  wr : Inport  Port=6
  Discrete-Time Integrator : DiscreteIntegrator  SampleTime=Ts  ICPrevOutput=DiscIntNeverNeededParam  ICPrevScaledInput=DiscIntNeverNeededParam
  a31 : Constant  Value=Rr*Lm/(Ls*Lr-Lm*Lm)
  a31*phisbeta_est : Product
  a33 : Constant  Value=-Rr*Ls/(Ls*Lr-Lm*Lm)
  a33*phirbeta_est : Product
  a34 caculation : Subsystem
  a34*phiralpha_est : Product
  dphirbeta_est/dt : Sum  Inputs=+-+++
  k1 : Constant  Value=(Rr*Ls+k*k*Rs*Lr-k*Rs*Lr-k*Rr*Ls)/Lm
  k3*(isbeta-isbeta_est) : Product
  k4 caculation : Subsystem
  k4*(isalpha-isalpha_est) : Product
  phirbeta_est2 : Outport
  wires:
  wr/1 -> k4 caculation/1(wr), a34 caculation/1(wr)
  dphirbeta_est/dt/1 -> Discrete-Time Integrator/1
  k3*(isbeta-isbeta_est)/1 -> dphirbeta_est/dt/5
  isbeta-isbeta_est/1 -> k3*(isbeta-isbeta_est)/2
  a31/1 -> a31*phisbeta_est/1
  a31*phisbeta_est/1 -> dphirbeta_est/dt/1
  a34 caculation/1(a34) -> a34*phiralpha_est/1
  k4*(isalpha-isalpha_est)/1 -> dphirbeta_est/dt/4
  a34*phiralpha_est/1 -> dphirbeta_est/dt/2
  Discrete-Time Integrator/1 -> phirbeta_est2/1
  phiralpha_est/1 -> a34*phiralpha_est/2
  isalpha-isalpha_est/1 -> k4*(isalpha-isalpha_est)/2
  phisbeta_est/1 -> a31*phisbeta_est/2
  k4 caculation/1(k4) -> k4*(isalpha-isalpha_est)/1
  a33*phirbeta_est/1 -> dphirbeta_est/dt/3
  a33/1 -> a33*phirbeta_est/1
  phirbeta_est/1 -> a33*phirbeta_est/2
  k1/1 -> k3*(isbeta-isbeta_est)/1

== system FullOrderObserver/FOO/full order flux observer/phisalpha_est caculation ==
  phisalpha_est : Inport
  phiralpha_est : Inport  Port=2
  usalpha : Inport  Port=3
  isalpha-isalpha_est : Inport  Port=4
  Discrete-Time Integrator : DiscreteIntegrator  SampleTime=Ts  ICPrevOutput=DiscIntNeverNeededParam  ICPrevScaledInput=DiscIntNeverNeededParam
  a11 : Constant  Value=-Rs*Lr/(Ls*Lr-Lm*Lm)
  a11*phisalpha_est : Product
  a13 : Constant  Value=Rs*Lm/(Ls*Lr-Lm*Lm)
  a13*phiralpha_est : Product
  dphisalpha_est/dt : Sum  Inputs=++++
  k1 : Constant  Value=Rs*(k*k-1)
  k1*(isalpha-isalpha_est) : Product
  phisalpha_est2 : Outport
  wires:
  a11/1 -> a11*phisalpha_est/1
  a11*phisalpha_est/1 -> dphisalpha_est/dt/1
  a13/1 -> a13*phiralpha_est/1
  k1*(isalpha-isalpha_est)/1 -> dphisalpha_est/dt/4
  usalpha/1 -> dphisalpha_est/dt/3
  a13*phiralpha_est/1 -> dphisalpha_est/dt/2
  Discrete-Time Integrator/1 -> phisalpha_est2/1
  dphisalpha_est/dt/1 -> Discrete-Time Integrator/1
  phiralpha_est/1 -> a13*phiralpha_est/2
  isalpha-isalpha_est/1 -> k1*(isalpha-isalpha_est)/2
  phisalpha_est/1 -> a11*phisalpha_est/2
  k1/1 -> k1*(isalpha-isalpha_est)/1

== system FullOrderObserver/FOO/full order flux observer/phisbeta_est caculation ==
  phisbeta_est : Inport
  phirbeta_est : Inport  Port=2
  usbeta : Inport  Port=3
  isbeta-isbeta_est : Inport  Port=4
  Discrete-Time Integrator : DiscreteIntegrator  SampleTime=Ts  ICPrevOutput=DiscIntNeverNeededParam  ICPrevScaledInput=DiscIntNeverNeededParam
  a11 : Constant  Value=-Rs*Lr/(Ls*Lr-Lm*Lm)
  a11*phisbeta_est : Product
  a13 : Constant  Value=Rs*Lm/(Ls*Lr-Lm*Lm)
  a13*phirbeta_est : Product
  dphisbeta_est/dt : Sum  Inputs=++++
  k1 : Constant  Value=Rs*(k*k-1)
  k1*(isbeta-isbeta_est) : Product
  phisbeta_est2 : Outport
  wires:
  k1/1 -> k1*(isbeta-isbeta_est)/1
  phisbeta_est/1 -> a11*phisbeta_est/2
  isbeta-isbeta_est/1 -> k1*(isbeta-isbeta_est)/2
  phirbeta_est/1 -> a13*phirbeta_est/2
  dphisbeta_est/dt/1 -> Discrete-Time Integrator/1
  Discrete-Time Integrator/1 -> phisbeta_est2/1
  a13*phirbeta_est/1 -> dphisbeta_est/dt/2
  usbeta/1 -> dphisbeta_est/dt/3
  k1*(isbeta-isbeta_est)/1 -> dphisbeta_est/dt/4
  a13/1 -> a13*phirbeta_est/1
  a11*phisbeta_est/1 -> dphisbeta_est/dt/1
  a11/1 -> a11*phisbeta_est/1

== system FullOrderObserver/SVPWM/SVPWM/N1 ==
  Ualfa : Inport
  Ubeta : Inport  Port=2
  Constant : Constant
  Constant1 : Constant  Value=0
  Gain : Gain  Gain=1.732
  Gain1 : Gain  Gain=-1.732
  Gain2 : Gain  Gain=2
  Gain3 : Gain  Gain=4
  Sum : Sum  Inputs=|-+
  Sum1 : Sum  Inputs=|-+
  Sum2 : Sum  Inputs=|+++
  Switch : Switch  SaturateOnIntegerOverflow=off  InputSameDT=off
  Switch1 : Switch  SaturateOnIntegerOverflow=off  InputSameDT=off
  Switch2 : Switch  SaturateOnIntegerOverflow=off  InputSameDT=off
  N : Outport
  wires:
  Ubeta/1 -> Switch/2, Sum1/1, Sum/1
  Constant/1 -> Switch/1, Switch2/1, Switch1/1
  Ualfa/1 -> Gain1/1, Gain/1
  Gain/1 -> Sum/2
  Sum/1 -> Switch1/2
  Sum1/1 -> Switch2/2
  Gain1/1 -> Sum1/2
  Constant1/1 -> Switch/3, Switch1/3, Switch2/3
  Switch1/1 -> Gain2/1
  Switch2/1 -> Gain3/1
  Gain2/1 -> Sum2/2
  Switch/1 -> Sum2/1
  Gain3/1 -> Sum2/3
  Sum2/1 -> N/1

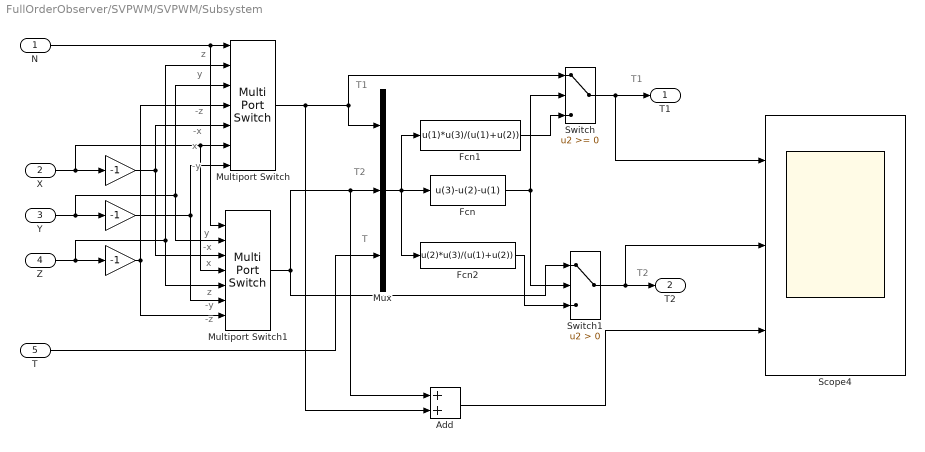
== system FullOrderObserver/SVPWM/SVPWM/Subsystem ==
  note: z
  note: y
  note: -z
  note: -x
  note: x
  note: -y
  note: y
  note: -x
  note: x
  note: z
  note: -y
  note: -z
  note: T1
  note: T2
  note: T
  note: T1
  note: T2
  N : Inport
  X : Inport  Port=2
  Y : Inport  Port=3
  Z : Inport  Port=4
  T : Inport  Port=5
  " " : Gain  Gain=-1
  "  " : Gain  Gain=-1
  "    " : Gain  Gain=-1
  Add : Sum
  Fcn : Fcn  Expr=u(3)-u(2)-u(1)
  Fcn1 : Fcn  Expr=u(1)*u(3)/(u(1)+u(2))
  Fcn2 : Fcn  Expr=u(2)*u(3)/(u(1)+u(2))
  Multiport Switch : MultiPortSwitch  Inputs=6  SaturateOnIntegerOverflow=off  InputSameDT=off
  Multiport Switch1 : MultiPortSwitch  Inputs=6  SaturateOnIntegerOverflow=off  InputSameDT=off
  Mux : Mux  Inputs=3
  Scope4 : Scope  NumInputPorts=3
  Switch : Switch  SaturateOnIntegerOverflow=off  InputSameDT=off
  Switch1 : Switch  Criteria=u2 > Threshold  SaturateOnIntegerOverflow=off  InputSameDT=off
  T1 : Outport
  T2 : Outport  Port=2
  wires:
  N/1 -> Multiport Switch1/1, Multiport Switch/1
  X/1 -> Multiport Switch1/4, Multiport Switch/6, " "/1
  Y/1 -> Multiport Switch1/2, Multiport Switch/3, "  "/1
  Z/1 -> Multiport Switch1/5, Multiport Switch/2, "    "/1
  "    "/1 -> Multiport Switch1/7, Multiport Switch/4
  "  "/1 -> Multiport Switch/7, Multiport Switch1/6
  " "/1 -> Multiport Switch/5, Multiport Switch1/3
  Multiport Switch/1 -> Switch/1, Mux/1, Add/2
  Multiport Switch1/1 -> Switch1/1, Mux/2, Add/1
  T/1 -> Mux/3
  Mux/1 -> Fcn/1, Fcn1/1, Fcn2/1
  Fcn/1 -> Switch/2, Switch1/2
  Fcn1/1 -> Switch/3
  Fcn2/1 -> Switch1/3
  Switch/1 -> T1/1, Scope4/1
  Switch1/1 -> T2/1, Scope4/2
  Add/1 -> Scope4/3

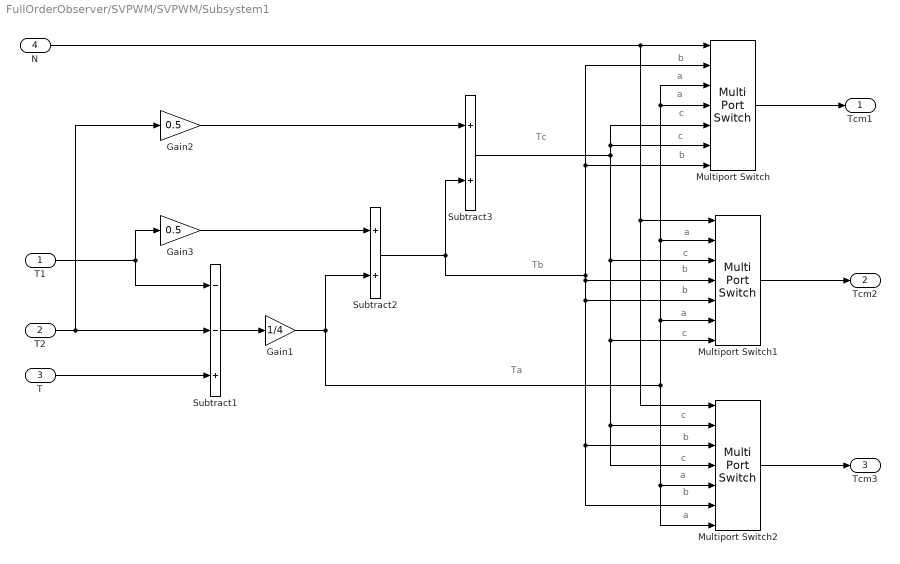
== system FullOrderObserver/SVPWM/SVPWM/Subsystem1 ==
  note: Ta
  note: Tb
  note: Tc
  note: b
  note: a
  note: a
  note: c
  note: c
  note: b
  note: a
  note: c
  note: b
  note: b
  note: a
  note: c
  note: c
  note: b
  note: c
  note: a
  note: b
  note: a
  T1 : Inport
  T2 : Inport  Port=2
  T : Inport  Port=3
  N : Inport  Port=4
  Gain1 : Gain  Gain=1/4
  Gain2 : Gain  Gain=0.5
  Gain3 : Gain  Gain=0.5
  Multiport Switch : MultiPortSwitch  Inputs=6  SaturateOnIntegerOverflow=off  InputSameDT=off
  Multiport Switch1 : MultiPortSwitch  Inputs=6  SaturateOnIntegerOverflow=off  InputSameDT=off
  Multiport Switch2 : MultiPortSwitch  Inputs=6  SaturateOnIntegerOverflow=off  InputSameDT=off
  Subtract1 : Sum  Inputs=--+
  Subtract2 : Sum
  Subtract3 : Sum
  Tcm1 : Outport
  Tcm2 : Outport  Port=2
  Tcm3 : Outport  Port=3
  wires:
  T2/1 -> Gain2/1, Subtract1/2
  T/1 -> Subtract1/3
  T1/1 -> Gain3/1, Subtract1/1
  Gain3/1 -> Subtract2/1
  Subtract1/1 -> Gain1/1
  Gain1/1 -> Subtract2/2, Multiport Switch/3, Multiport Switch/4, Multiport Switch1/2, Multiport Switch1/6, Multiport Switch2/5, Multiport Switch2/7
  Subtract2/1 -> Multiport Switch/2, Multiport Switch/7, Multiport Switch1/4, Multiport Switch1/5, Multiport Switch2/3, Multiport Switch2/6, Subtract3/2
  Gain2/1 -> Subtract3/1
  N/1 -> Multiport Switch/1, Multiport Switch2/1, Multiport Switch1/1
  Multiport Switch/1 -> Tcm1/1
  Multiport Switch1/1 -> Tcm2/1
  Multiport Switch2/1 -> Tcm3/1
  Subtract3/1 -> Multiport Switch/5, Multiport Switch/6, Multiport Switch1/3, Multiport Switch1/7, Multiport Switch2/2, Multiport Switch2/4

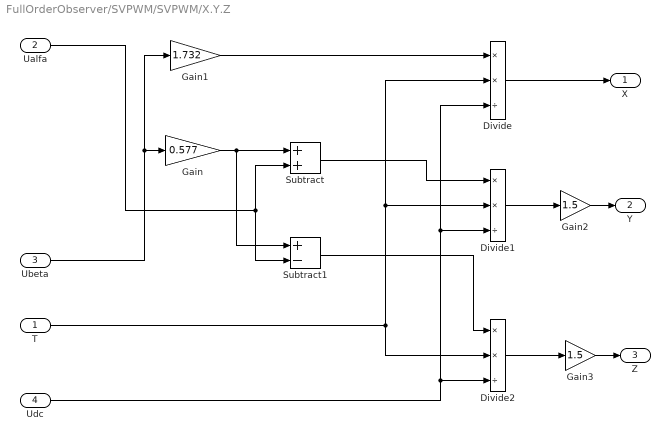
== system FullOrderObserver/SVPWM/SVPWM/X.Y.Z ==
  T : Inport
  Ualfa : Inport  Port=2
  Ubeta : Inport  Port=3
  Udc : Inport  Port=4
  Divide : Product  Inputs=**/
  Divide1 : Product  Inputs=**/
  Divide2 : Product  Inputs=**/
  Gain : Gain  Gain=0.577
  Gain1 : Gain  Gain=1.732
  Gain2 : Gain  Gain=1.5
  Gain3 : Gain  Gain=1.5
  Subtract : Sum
  Subtract1 : Sum  Inputs=+-
  X : Outport
  Y : Outport  Port=2
  Z : Outport  Port=3
  wires:
  Gain/1 -> Subtract/1, Subtract1/1
  Gain1/1 -> Divide/1
  T/1 -> Divide2/2, Divide1/2, Divide/2
  Udc/1 -> Divide2/3, Divide1/3, Divide/3
  Ualfa/1 -> Subtract1/2, Subtract/2
  Subtract/1 -> Divide1/1
  Subtract1/1 -> Divide2/1
  Divide/1 -> X/1
  Divide1/1 -> Gain2/1
  Divide2/1 -> Gain3/1
  Gain2/1 -> Y/1
  Gain3/1 -> Z/1
  Ubeta/1 -> Gain/1, Gain1/1

== system FullOrderObserver/FOO/full order flux observer/phiralpha_est caculation/a34 caculation ==
  wr : Inport
  -wr : Gain  Gain=-1
  a34 : Outport
  wires:
  wr/1 -> -wr/1
  -wr/1 -> a34/1

== system FullOrderObserver/FOO/full order flux observer/phiralpha_est caculation/k4 caculation ==
  wr : Inport
  ((k-1)*(Ls*Lr-Lm*Lm))/Lm : Constant  Value=((k-1)*(Ls*Lr-Lm*Lm))/Lm
  Product : Product
  k4 : Outport
  wires:
  Product/1 -> k4/1
  wr/1 -> Product/1
  ((k-1)*(Ls*Lr-Lm*Lm))/Lm/1 -> Product/2

== system FullOrderObserver/FOO/full order flux observer/phirbeta_est caculation/a34 caculation ==
  wr : Inport
  -wr : Gain  Gain=-1
  a34 : Outport
  wires:
  wr/1 -> -wr/1
  -wr/1 -> a34/1

== system FullOrderObserver/FOO/full order flux observer/phirbeta_est caculation/k4 caculation ==
  wr : Inport
  ((k-1)*(Ls*Lr-Lm*Lm))/Lm : Constant  Value=((k-1)*(Ls*Lr-Lm*Lm))/Lm
  Product : Product
  k4 : Outport
  wires:
  ((k-1)*(Ls*Lr-Lm*Lm))/Lm/1 -> Product/2
  wr/1 -> Product/1
  Product/1 -> k4/1
